simulink model "lab04z4_sch"  (Simulink 9.0)
settings: Solver=ode3  StartTime=0.0  StopTime=10  FixedStep=0.001  RelTol=1e-3  EnableMultiTasking=on
InitFcn:
  | clear all; close all;
  | % Parametry obiektu
  | R = 3;
  | L = 0.05;
  | kfi = 2.23;
  | J = 0.11;
  | % Obserwator
  | Lo = [-44.6, 60];
  | % Sprzezenie od stanu
  | K1 = [ 0.0, 0.010269058295964];
  | K2 = [-2.1, 0.096591928251121];
settings Model: Creator=Jacek  LastModifiedBy=Jacek
settings DataIOCC: LimitDataPoints=on
settings DebuggingCC: UnderspecifiedInitializationDetection=Simplified  MergeDetectMultiDrivingBlocksExec=error  SolverPrmCheckMsg=warning
settings GRTTargetCC: GeneratePreprocessorConditionals=Disable all
settings ConfigComp: CovSFcnEnable=off

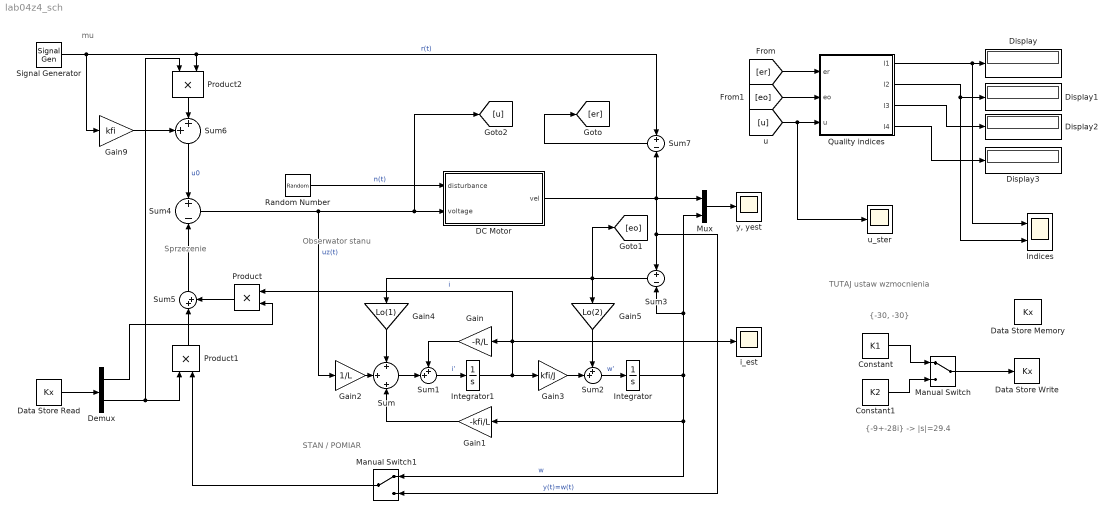
== system lab04z4_sch ==
  note: STAN / POMIAR
  note: TUTAJ ustaw wzmocnienia
  note: {-30, -30}
  note: mu
  note: Obserwator stanu
  note: Sprzezenie
  note: {-9+-28i} -> |s|=29.4
  Constant : Constant  Value=K1
  Constant1 : Constant  Value=K2
  DC Motor : Subsystem
  Data Store Memory : DataStoreMemory  DataStoreName=Kx  ReadBeforeWriteMsg=warning  WriteAfterWriteMsg=warning  WriteAfterReadMsg=warning  InitialValue=[0, 0]  ShowAdditionalParam=off
  Data Store Read : DataStoreRead  DataStoreName=Kx
  Data Store Write : DataStoreWrite  DataStoreName=Kx
  Demux : Demux  Outputs=2
  Display{,1..3} (4 alike) : Display
  Gain : Gain  Gain=-R/L
  Gain1 : Gain  Gain=-kfi/L
  Gain2 : Gain  Gain=1/L
  Gain3 : Gain  Gain=kfi/J
  Gain4 : Gain  Gain=Lo(1)
  Gain5 : Gain  Gain=Lo(2)
  Gain9 : Gain  Gain=kfi
  Indices : Scope  NumInputPorts=2
  Integrator : Integrator
  Integrator1 : Integrator
  Manual Switch : ManualSwitch
  Manual Switch1 : ManualSwitch
  Mux : Mux  Inputs=2
  Product : Product
  Product1 : Product
  Product2 : Product
  Quality indices : Subsystem
  Random Number : RandomNumber  Variance=1e-3
  Signal Generator : SignalGenerator  WaveForm=square  Frequency=0.5
  Sum : Sum  Inputs=+|+|+
  Sum1 : Sum  Inputs=++|
  Sum2 : Sum  Inputs=++|
  Sum3 : Sum  Inputs=+|-
  Sum4 : Sum  Inputs=+|-
  Sum5 : Sum  Inputs=|++
  Sum6 : Sum  Inputs=++|
  Sum7 : Sum  Inputs=+|-
  i_est : Scope
  u_ster : Scope
  "y, yest" : Scope
  wires:
  Random Number/1 -> DC Motor/1(disturbance)  "n(t)"
  Sum4/1 -> Gain2/1, [u], DC Motor/2(voltage)  "uz(t)"
  DC Motor/1(vel) -> Manual Switch1/2, Sum3/1, Sum7/2, Mux/1  "y(t)=w(t)"
  Gain2/1 -> Sum/2
  Sum1/1 -> Integrator1/1  "i'"
  Gain/1 -> Sum1/1
  Sum/1 -> Sum1/2
  Gain1/1 -> Sum/3
  Sum2/1 -> Integrator/1  "w'"
  Gain3/1 -> Sum2/2
  Sum3/1 -> [eo], Gain5/1, Gain4/1
  Gain5/1 -> Sum2/1
  Gain4/1 -> Sum/1
  Mux/1 -> "y, yest"/1
  Integrator/1 -> Manual Switch1/1, Gain1/1, Sum3/2, Mux/2  "w"
  Product/1 -> Sum5/2
  Sum5/1 -> Sum4/2
  Product1/1 -> Sum5/1
  Integrator1/1 -> Product/1, i_est/1, Gain/1, Gain3/1  "i"
  Sum6/1 -> Sum4/1  "u0"
  Gain9/1 -> Sum6/1
  Product2/1 -> Sum6/2
  Signal Generator/1 -> Product2/2, Sum7/1, Gain9/1  "r(t)"
  Sum7/1 -> [er]
  Quality indices/4(I4) -> Display3/1
  Quality indices/1(I1) -> Indices/1, Display/1
  Quality indices/2(I2) -> Display1/1, Indices/2
  Quality indices/3(I3) -> Display2/1
  [er] -> Quality indices/1(er)
  [eo] -> Quality indices/2(eo)
  [u] -> u_ster/1, Quality indices/3(u)
  Constant/1 -> Manual Switch/1
  Constant1/1 -> Manual Switch/2
  Manual Switch/1 -> Data Store Write/1
  Data Store Read/1 -> Demux/1
  Demux/1 -> Product/2
  Demux/2 -> Product2/1, Product1/1
  Manual Switch1/1 -> Product1/2

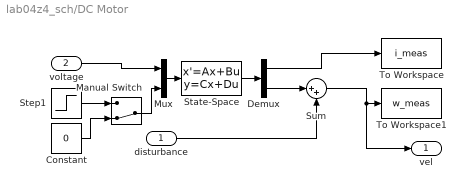
== system lab04z4_sch/DC Motor ==
  disturbance : Inport
  voltage : Inport  Port=2
  Constant : Constant  Value=0
  Demux : Demux  Outputs=2
  Manual Switch : ManualSwitch  CurrentSetting=0
  Mux : Mux  Inputs=2
  State-Space : StateSpace  A=[-3/0.05, -2.23/0.05; 2.23/0.11, 0]  B=[1/0.05 0; 0 -1/0.11]  C=[1 0;0 1]  D=[0 0; 0 0]  InitialCondition=[0 ;0]
  Step1 : Step  Time=0.5  After=44.6*1  SampleTime=0
  Sum : Sum  Inputs=|++
  To Workspace : ToWorkspace  VariableName=i_meas  SampleTime=-1
  To Workspace1 : ToWorkspace  VariableName=w_meas  SampleTime=-1
  vel : Outport
  wires:
  Mux/1 -> State-Space/1
  voltage/1 -> Mux/1
  Step1/1 -> Manual Switch/1
  State-Space/1 -> Demux/1
  Demux/1 -> To Workspace/1
  disturbance/1 -> Sum/2
  Sum/1 -> vel/1, To Workspace1/1
  Demux/2 -> Sum/1
  Manual Switch/1 -> Mux/2
  Constant/1 -> Manual Switch/2

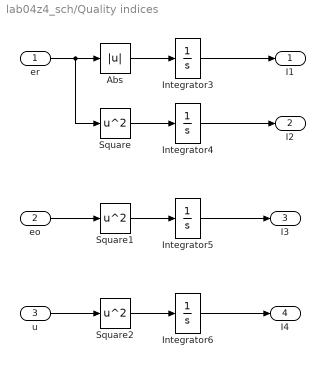
== system lab04z4_sch/Quality indices ==
  er : Inport
  eo : Inport  Port=2
  u : Inport  Port=3
  Abs : Abs
  Integrator{3..6} (4 alike) : Integrator
  Square : Math  Operator=square  RndMeth=Zero  SaturateOnIntegerOverflow=on
  Square1 : Math  Operator=square  RndMeth=Zero  SaturateOnIntegerOverflow=on
  Square2 : Math  Operator=square  RndMeth=Zero  SaturateOnIntegerOverflow=on
  I1 : Outport
  I2 : Outport  Port=2
  I3 : Outport  Port=3
  I4 : Outport  Port=4
  wires:
  eo/1 -> Square1/1
  Square2/1 -> Integrator6/1
  Integrator6/1 -> I4/1
  u/1 -> Square2/1
  er/1 -> Abs/1, Square/1
  Integrator4/1 -> I2/1
  Square1/1 -> Integrator5/1
  Integrator5/1 -> I3/1
  Abs/1 -> Integrator3/1
  Integrator3/1 -> I1/1
  Square/1 -> Integrator4/1
